simulink model "SVPWM"  (R2023a)
settings: Solver=VariableStepAuto  StartTime=0.0  StopTime=1  MaxStep=0.0001  RelTol=1e-3
libraries: spsMosfetLib x6, spspowerguiLib x2, spsThreePhaseVIMeasurementLib x2, spsDCVoltageSourceLib x1, spsGroundLib x1, spsThreePhaseSeriesRLCBranchLib x1, spsTriangleGeneratorLib x1
settings Model: Creator=patri  LastModifiedBy=patri

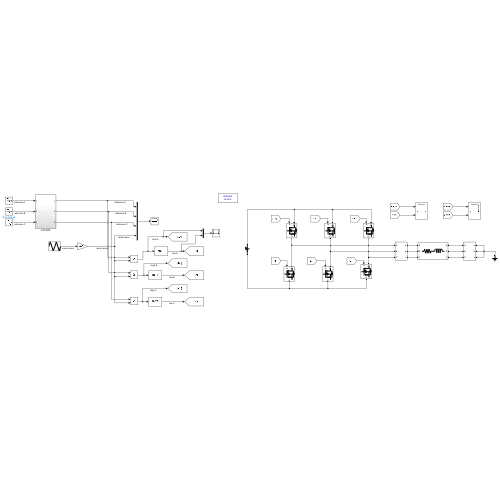
[thumbnail: Simulink's stored preview of the top-level diagram]
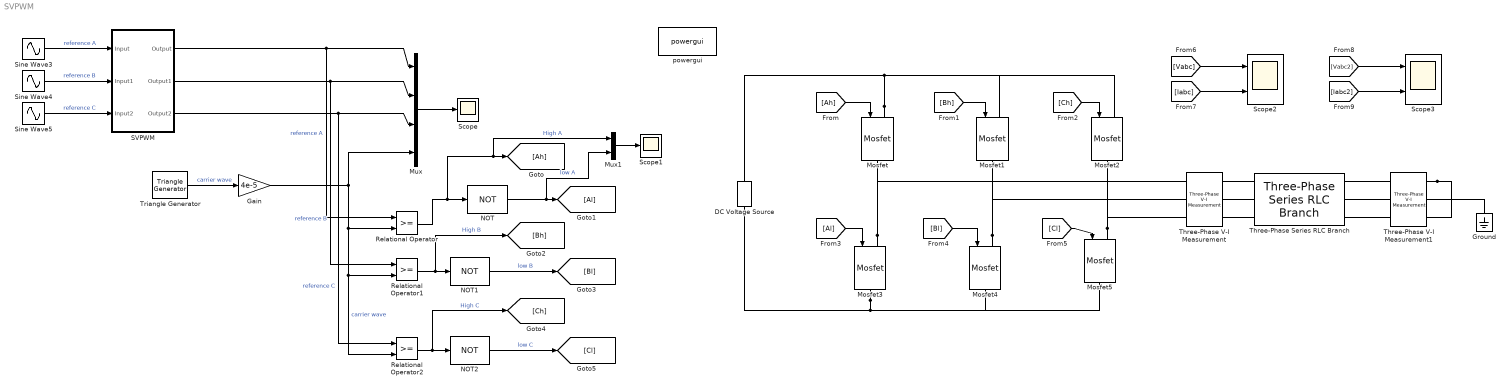
== system SVPWM ==
  DC Voltage Source : spsDCVoltageSourceLib/DC Voltage Source  Amplitude=100  Measurements=None
  Gain : Gain  Gain=4e-5
  Ground : spsGroundLib/Ground  LConnTagsString=a
  Mosfet{,1..5} (6 alike) : spsMosfetLib/Mosfet  Ron=0.1  Lon=0  Rd=0.01  Vfd=0  IC=0  Rs=1e5  Cs=inf  Measurements=off
  Mux : Mux
  Mux1 : Mux  Inputs=2
  NOT : Logic  Operator=NOT  AllPortsSameDT=off  OutDataTypeStr=boolean
  NOT1 : Logic  Operator=NOT  AllPortsSameDT=off  OutDataTypeStr=boolean
  NOT2 : Logic  Operator=NOT  AllPortsSameDT=off  OutDataTypeStr=boolean
  Relational Operator : RelationalOperator  OutDataTypeStr=boolean  RndMeth=Simplest  InputSameDT=off
  Relational Operator1 : RelationalOperator  OutDataTypeStr=boolean  RndMeth=Simplest  InputSameDT=off
  Relational Operator2 : RelationalOperator  OutDataTypeStr=boolean  RndMeth=Simplest  InputSameDT=off
  SVPWM : Subsystem
  Scope : Scope
  Scope1 : Scope
  Scope2 : Scope  NumInputPorts=2
  Scope3 : Scope  NumInputPorts=2
  Sine Wave3 : Sin  Frequency=2*pi*50  SampleTime=0
  Sine Wave4 : Sin  Frequency=2*pi*50  Phase=2*pi/3  SampleTime=0
  Sine Wave5 : Sin  Frequency=2*pi*50  Phase=4*pi/3  SampleTime=0
  Three-Phase Series RLC Branch : spsThreePhaseSeriesRLCBranchLib/Three-Phase Series RLC Branch  LConnTagsString=A|B|C  RConnTagsString=A|B|C  BranchType=RL  Resistance=1  Inductance=1e-3  Capacitance=1e-6  Measurements=None
  Three-Phase V-I Measurement : spsThreePhaseVIMeasurementLib/Three-Phase V-I Measurement  VoltageMeasurement=phase-to-ground  SetLabelV=on  LabelV=Vabc  Vpu=off  VpuLL=off  CurrentMeasurement=yes  SetLabelI=on  LabelI=Iabc  Ipu=off  Pbase=100e6  Vbase=500e3  OutputType=Complex  PhasorSimulation=off  PSBequivalent=0
  Three-Phase V-I Measurement1 : spsThreePhaseVIMeasurementLib/Three-Phase V-I Measurement  VoltageMeasurement=phase-to-ground  SetLabelV=on  LabelV=Vabc2  Vpu=off  VpuLL=off  CurrentMeasurement=yes  SetLabelI=on  LabelI=Iabc2  Ipu=off  Pbase=100e6  Vbase=500e3  OutputType=Complex  PhasorSimulation=off  PSBequivalent=0
  Triangle Generator : spsTriangleGeneratorLib/Triangle Generator  Freq=10e3  Phase=90  Ts=0
  powergui : spspowerguiLib/powergui  Priority=1  SimulationMode=Discrete  SampleTime=1e-6  frequency=60  Iterations=50  frequencyindice=0  Pbase=100e6  ErrMax=1e-4  UnitsV=kV  UnitsW=MW  buscounter=0  FunctionMessages=off  echomessages=off  EnableUseOfTLC=off  CurrentSourceSwitches=off  DisableSnubberDevices=off  DisableRonSwitches=off  DisableVfSwitches=off  DisplayEquations=off  AutomaticDiscreteSolvers=off  SolverType=Tustin/Backward Euler (TBE)  Interpol=off  ExternalGateDelay=off  methode=off  Ts=100  x0status=blocks  SPID=on  SwTol=0  HookPort=off  NonlinearTolerance=1e-4  nMaxIteration=100  ContinueOnMaxIteration=off  RestoreLinks=warning  ResistiveCurrentMeasurement=off  Frange=[0:2:500]  Ylog=off  Xlog=on  ShowGrid=off  save=off  variable=ZData  structure=0  ZoomFFT=off  StartTime=0.0  cycles=1  DisplayStyle=1  fundamental=60  FreqAxis=off  MaxFrequency=1000  frequencyindicesteady=1  RmsSteady=1  display=off
  wires:
  [Vabc2] -> Scope3/1
  [Al] -> Mosfet3/1
  [Vabc] -> Scope2/1
  [Cl] -> Mosfet5/1
  [Bh] -> Mosfet1/1
  [Ch] -> Mosfet2/1
  [Bl] -> Mosfet4/1
  [Iabc] -> Scope2/2
  [Iabc2] -> Scope3/2
  [Ah] -> Mosfet/1
  Sine Wave3/1 -> SVPWM/1(Input)  "reference A"
  Sine Wave4/1 -> SVPWM/2(Input1)  "reference B"
  Sine Wave5/1 -> SVPWM/3(Input2)  "reference C"
  Mux/1 -> Scope/1
  Mux1/1 -> Scope1/1
  NOT1/1 -> [Bl]  "low B"
  NOT/1 -> Mux1/2, [Al]  "low A"
  Relational Operator2/1 -> [Ch], NOT2/1  "High C"
  NOT2/1 -> [Cl]  "low C"
  Triangle Generator/1 -> Gain/1  "carrier wave"
  Relational Operator1/1 -> [Bh], NOT1/1  "High B"
  Relational Operator/1 -> Mux1/1, [Ah], NOT/1  "High A"
  SVPWM/3(Output2) -> Relational Operator2/1, Mux/3  "reference C"
  SVPWM/2(Output1) -> Relational Operator1/1, Mux/2  "reference B"
  SVPWM/1(Output) -> Relational Operator/1, Mux/1  "reference A"
  Gain/1 -> Relational Operator2/2, Relational Operator1/2, Relational Operator/2, Mux/4  "carrier wave"
  connections:
  Mosfet3/RConn1 -- DC Voltage Source/LConn1 -- Mosfet4/RConn1 -- Mosfet5/RConn1
  Three-Phase V-I Measurement1/RConn1 -- Three-Phase V-I Measurement1/RConn2 -- Ground/LConn1 -- Three-Phase V-I Measurement1/RConn3
  Mosfet/LConn1 -- DC Voltage Source/RConn1 -- Mosfet2/LConn1 -- Mosfet1/LConn1
  Mosfet4/LConn1 -- Mosfet1/RConn1 -- Three-Phase V-I Measurement/LConn2
  Mosfet3/LConn1 -- Mosfet/RConn1 -- Three-Phase V-I Measurement/LConn1
  Mosfet5/LConn1 -- Mosfet2/RConn1 -- Three-Phase V-I Measurement/LConn3
  Three-Phase V-I Measurement/RConn1 -- Three-Phase Series RLC Branch/LConn1
  Three-Phase V-I Measurement1/LConn3 -- Three-Phase Series RLC Branch/RConn3
  Three-Phase V-I Measurement1/LConn1 -- Three-Phase Series RLC Branch/RConn1
  Three-Phase Series RLC Branch/LConn2 -- Three-Phase V-I Measurement/RConn2
  Three-Phase V-I Measurement/RConn3 -- Three-Phase Series RLC Branch/LConn3
  Three-Phase V-I Measurement1/LConn2 -- Three-Phase Series RLC Branch/RConn2

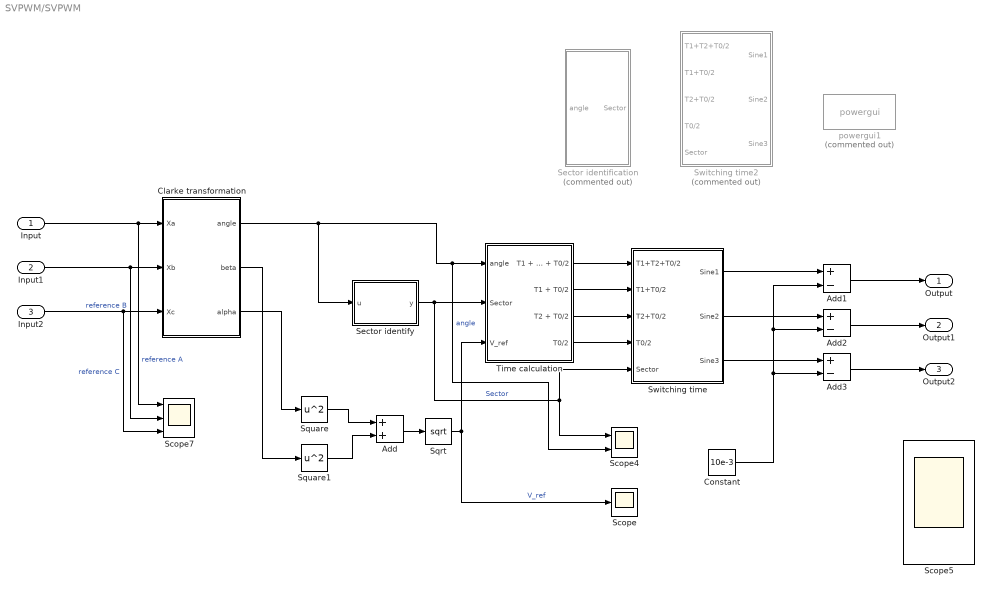
== system SVPWM/SVPWM ==
  Input : Inport
  Input1 : Inport  Port=2
  Input2 : Inport  Port=3
  Add : Sum
  Add1 : Sum  Inputs=+-
  Add2 : Sum  Inputs=+-
  Add3 : Sum  Inputs=+-
  Clarke transformation : Subsystem
  Constant : Constant  Value=10e-3
  Scope : Scope
  Scope4 : Scope  NumInputPorts=2
  Scope5 : Scope  NumInputPorts=3
  Scope7 : Scope  NumInputPorts=3
  Sector identification : Subsystem  Commented=on
  Sector identify : MATLAB Function  TreatAsAtomicUnit=on
  Sqrt : Sqrt
  Square : Math  Operator=square
  Square1 : Math  Operator=square
  Switching time : Subsystem
  Switching time2 : Subsystem  Commented=on
  Time calculation : Subsystem
  powergui1 : spspowerguiLib/powergui  Priority=1  Commented=on  SimulationMode=Continuous  SampleTime=50e-6  frequency=60  Iterations=50  frequencyindice=60  Pbase=100e6  ErrMax=1e-4  UnitsV=kV  UnitsW=MW  buscounter=0  FunctionMessages=off  echomessages=off  EnableUseOfTLC=off  CurrentSourceSwitches=off  DisableSnubberDevices=off  DisableRonSwitches=off  DisableVfSwitches=off  DisplayEquations=off  AutomaticDiscreteSolvers=off  SolverType=Tustin/Backward Euler (TBE)  Interpol=off  ExternalGateDelay=off  methode=off  Ts=100  x0status=blocks  SPID=on  SwTol=0  HookPort=off  NonlinearTolerance=1e-4  nMaxIteration=100  ContinueOnMaxIteration=off  RestoreLinks=warning  ResistiveCurrentMeasurement=off  Frange=[0:2:500]  Ylog=off  Xlog=on  ShowGrid=off  save=off  variable=ZData  structure=0  ZoomFFT=off  StartTime=0.0  cycles=1  DisplayStyle=1  fundamental=60  FreqAxis=off  MaxFrequency=1000  frequencyindicesteady=1  RmsSteady=1  display=off
  Output : Outport
  Output1 : Outport  Port=2
  Output2 : Outport  Port=3
  wires:
  Sector identify/1(y) -> Switching time/5(Sector), Scope4/1, Time calculation/2(Sector)  "Sector"
  Sqrt/1 -> Scope/1, Time calculation/3(V_ref)  "V_ref"
  Input1/1 -> Scope7/2, Clarke transformation/2(Xb)  "reference B"
  Time calculation/3(T2 + T0/2) -> Switching time/3(T2+T0/2)
  Square/1 -> Add/1
  Square1/1 -> Add/2
  Time calculation/1(T1 + T2 + T0/2) -> Switching time/1(T1+T2+T0/2)
  Time calculation/2(T1 + T0/2) -> Switching time/2(T1+T0/2)
  Input/1 -> Scope7/1, Clarke transformation/1(Xa)  "reference A"
  Input2/1 -> Scope7/3, Clarke transformation/3(Xc)  "reference C"
  Clarke transformation/1(angle) -> Scope4/2, Time calculation/1(angle), Sector identify/1(u)  "angle"
  Time calculation/4(T0/2) -> Switching time/4(T0/2)
  Clarke transformation/2(beta) -> Square1/1
  Clarke transformation/3(alpha) -> Square/1
  Add/1 -> Sqrt/1
  Constant/1 -> Add3/2, Add2/2, Add1/2
  Switching time/1(Sine1) -> Add1/1
  Add1/1 -> Output/1
  Switching time/2(Sine2) -> Add2/1
  Switching time/3(Sine3) -> Add3/1
  Add2/1 -> Output1/1
  Add3/1 -> Output2/1

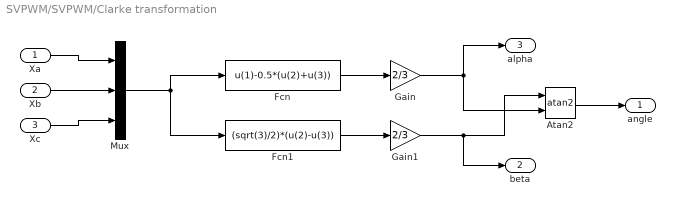
== system SVPWM/SVPWM/Clarke transformation ==
  Xa : Inport
  Xb : Inport  Port=2
  Xc : Inport  Port=3
  Atan2 : Trigonometry  Operator=atan2
  Fcn : Fcn  Expr=u(1)-0.5*(u(2)+u(3))
  Fcn1 : Fcn  Expr=(sqrt(3)/2)*(u(2)-u(3))
  Gain : Gain  Gain=2/3
  Gain1 : Gain  Gain=2/3
  Mux : Mux  Inputs=3
  angle : Outport
  beta : Outport  Port=2
  alpha : Outport  Port=3
  wires:
  Xc/1 -> Mux/3
  Xb/1 -> Mux/2
  Xa/1 -> Mux/1
  Mux/1 -> Fcn1/1, Fcn/1
  Fcn/1 -> Gain/1
  Fcn1/1 -> Gain1/1
  Gain/1 -> Atan2/2, alpha/1
  Gain1/1 -> Atan2/1, beta/1
  Atan2/1 -> angle/1

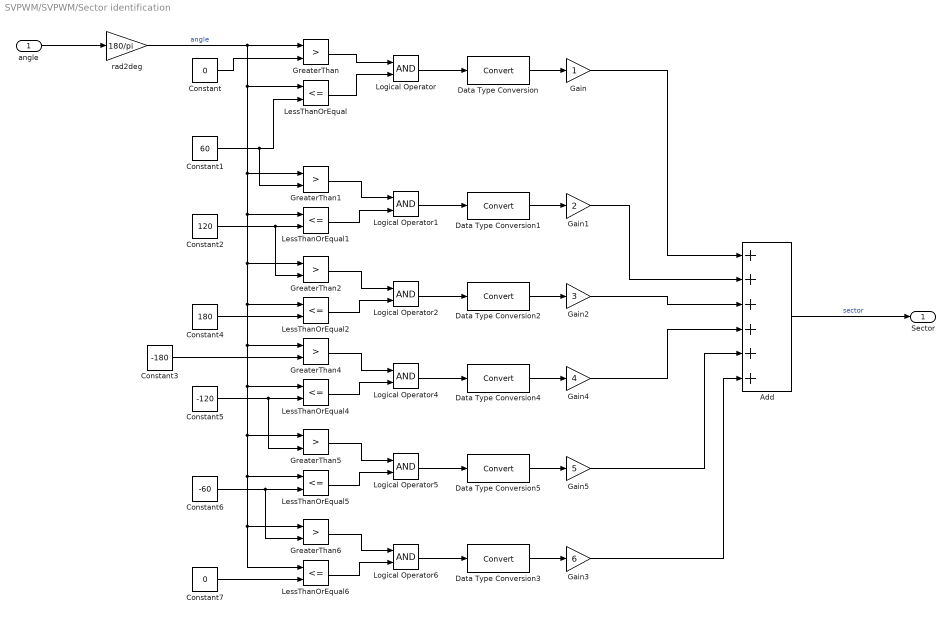
== system SVPWM/SVPWM/Sector identification ==
  angle : Inport
  Add : Sum  Inputs=++++++
  Constant : Constant  Value=0
  Constant1 : Constant  Value=60
  Constant2 : Constant  Value=120
  Constant3 : Constant  Value=-180
  Constant4 : Constant  Value=180
  Constant5 : Constant  Value=-120
  Constant6 : Constant  Value=-60
  Constant7 : Constant  Value=0
  Data Type Conversion{,1..5} (6 alike) : DataTypeConversion  SaturateOnIntegerOverflow=off  RndMeth=Floor
  Gain : Gain
  Gain1 : Gain  Gain=2
  Gain2 : Gain  Gain=3
  Gain3 : Gain  Gain=6
  Gain4 : Gain  Gain=4
  Gain5 : Gain  Gain=5
  GreaterThan{,1..2,4..6} (6 alike) : RelationalOperator  Operator=>  OutDataTypeStr=boolean  RndMeth=Simplest  InputSameDT=off
  LessThanOrEqual{,1..2,4..6} (6 alike) : RelationalOperator  Operator=<=  OutDataTypeStr=boolean  RndMeth=Simplest  InputSameDT=off
  Logical Operator{,1..2,4..6} (6 alike) : Logic  AllPortsSameDT=off  OutDataTypeStr=boolean
  rad2deg : Gain  Gain=180/pi
  Sector : Outport
  wires:
  Data Type Conversion1/1 -> Gain1/1
  LessThanOrEqual6/1 -> Logical Operator6/2
  Constant1/1 -> GreaterThan1/2, LessThanOrEqual/2
  LessThanOrEqual2/1 -> Logical Operator2/2
  LessThanOrEqual4/1 -> Logical Operator4/2
  LessThanOrEqual5/1 -> Logical Operator5/2
  Constant2/1 -> GreaterThan2/2, LessThanOrEqual1/2
  LessThanOrEqual/1 -> Logical Operator/2
  Constant7/1 -> LessThanOrEqual6/2
  Constant6/1 -> GreaterThan6/2, LessThanOrEqual5/2
  LessThanOrEqual1/1 -> Logical Operator1/2
  Constant4/1 -> LessThanOrEqual2/2
  GreaterThan5/1 -> Logical Operator5/1
  GreaterThan6/1 -> Logical Operator6/1
  GreaterThan4/1 -> Logical Operator4/1
  Data Type Conversion/1 -> Gain/1
  Data Type Conversion3/1 -> Gain3/1
  Logical Operator6/1 -> Data Type Conversion3/1
  Data Type Conversion4/1 -> Gain4/1
  Logical Operator2/1 -> Data Type Conversion2/1
  Constant5/1 -> GreaterThan5/2, LessThanOrEqual4/2
  Logical Operator4/1 -> Data Type Conversion4/1
  GreaterThan/1 -> Logical Operator/1
  Constant/1 -> GreaterThan/2
  GreaterThan1/1 -> Logical Operator1/1
  Logical Operator5/1 -> Data Type Conversion5/1
  Logical Operator/1 -> Data Type Conversion/1
  GreaterThan2/1 -> Logical Operator2/1
  Data Type Conversion5/1 -> Gain5/1
  Data Type Conversion2/1 -> Gain2/1
  Constant3/1 -> GreaterThan4/2
  Logical Operator1/1 -> Data Type Conversion1/1
  Gain/1 -> Add/1
  Gain1/1 -> Add/2
  Gain2/1 -> Add/3
  Gain4/1 -> Add/4
  Gain5/1 -> Add/5
  Gain3/1 -> Add/6
  Add/1 -> Sector/1  "sector"
  angle/1 -> rad2deg/1
  rad2deg/1 -> LessThanOrEqual6/1, GreaterThan6/1, LessThanOrEqual5/1, GreaterThan5/1, LessThanOrEqual4/1, GreaterThan4/1, LessThanOrEqual2/1, GreaterThan2/1, LessThanOrEqual1/1, GreaterThan1/1, LessThanOrEqual/1, GreaterThan/1  "angle"

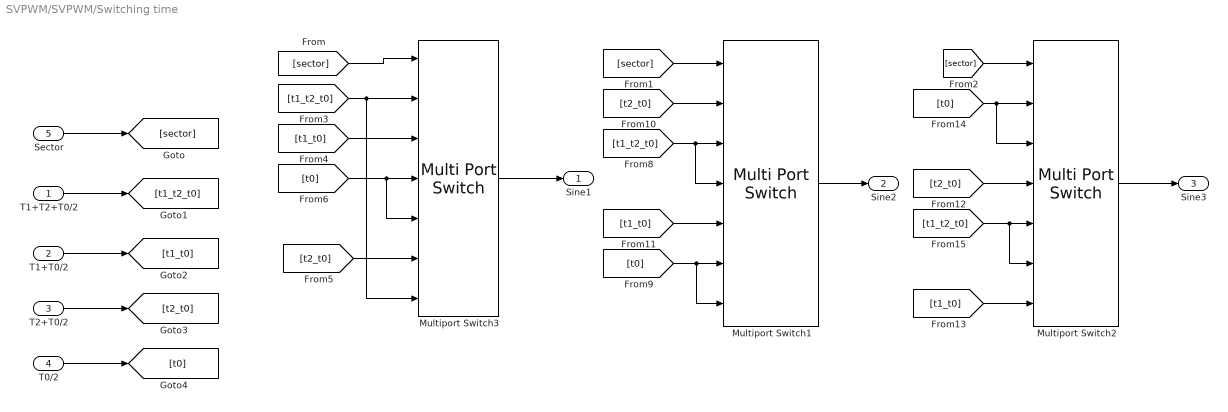
== system SVPWM/SVPWM/Switching time ==
  T1+T2+T0/2 : Inport
  T1+T0/2 : Inport  Port=2
  T2+T0/2 : Inport  Port=3
  T0/2 : Inport  Port=4
  Sector : Inport  Port=5
  Multiport Switch1 : MultiPortSwitch  Inputs=6  DiagnosticForDefault=Warning  SaturateOnIntegerOverflow=off  InputSameDT=off
  Multiport Switch2 : MultiPortSwitch  Inputs=6  DiagnosticForDefault=Warning  SaturateOnIntegerOverflow=off  InputSameDT=off
  Multiport Switch3 : MultiPortSwitch  Inputs=6  DiagnosticForDefault=Warning  SaturateOnIntegerOverflow=off  InputSameDT=off
  Sine1 : Outport
  Sine2 : Outport  Port=2
  Sine3 : Outport  Port=3
  wires:
  Multiport Switch3/1 -> Sine1/1
  Sector/1 -> [sector]
  T1+T2+T0/2/1 -> [t1_t2_t0]
  [sector] -> Multiport Switch3/1
  [sector] -> Multiport Switch1/1
  [sector] -> Multiport Switch2/1
  Multiport Switch1/1 -> Sine2/1
  Multiport Switch2/1 -> Sine3/1
  T1+T0/2/1 -> [t1_t0]
  T2+T0/2/1 -> [t2_t0]
  T0/2/1 -> [t0]
  [t1_t2_t0] -> Multiport Switch3/7, Multiport Switch3/2
  [t1_t2_t0] -> Multiport Switch1/4, Multiport Switch1/3
  [t1_t2_t0] -> Multiport Switch2/6, Multiport Switch2/5
  [t1_t0] -> Multiport Switch3/3
  [t0] -> Multiport Switch3/5, Multiport Switch3/4
  [t2_t0] -> Multiport Switch3/6
  [t2_t0] -> Multiport Switch1/2
  [t1_t0] -> Multiport Switch1/5
  [t0] -> Multiport Switch1/7, Multiport Switch1/6
  [t1_t0] -> Multiport Switch2/7
  [t2_t0] -> Multiport Switch2/4
  [t0] -> Multiport Switch2/3, Multiport Switch2/2

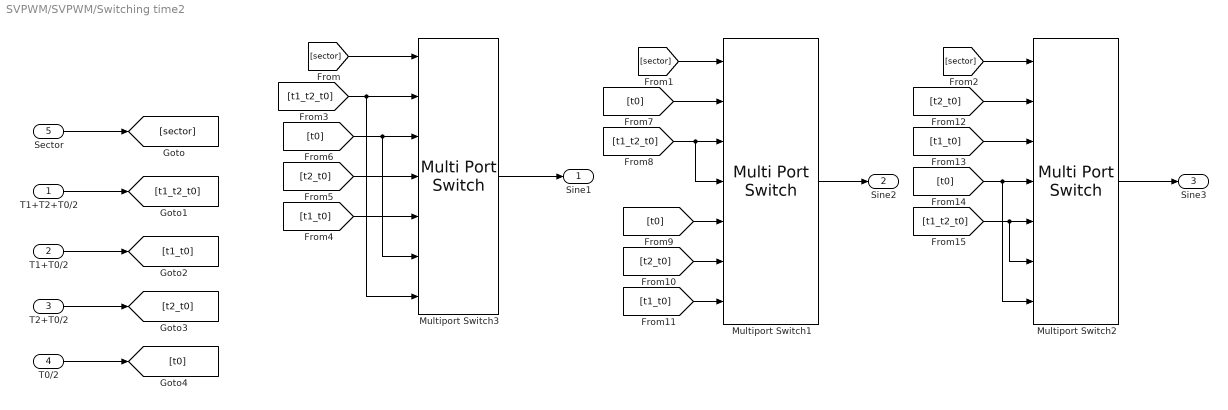
== system SVPWM/SVPWM/Switching time2 ==
  T1+T2+T0/2 : Inport
  T1+T0/2 : Inport  Port=2
  T2+T0/2 : Inport  Port=3
  T0/2 : Inport  Port=4
  Sector : Inport  Port=5
  Multiport Switch1 : MultiPortSwitch  Inputs=6  SaturateOnIntegerOverflow=off  InputSameDT=off
  Multiport Switch2 : MultiPortSwitch  Inputs=6  SaturateOnIntegerOverflow=off  InputSameDT=off
  Multiport Switch3 : MultiPortSwitch  Inputs=6  SaturateOnIntegerOverflow=off  InputSameDT=off
  Sine1 : Outport
  Sine2 : Outport  Port=2
  Sine3 : Outport  Port=3
  wires:
  Multiport Switch3/1 -> Sine1/1
  Sector/1 -> [sector]
  T1+T2+T0/2/1 -> [t1_t2_t0]
  [sector] -> Multiport Switch3/1
  [sector] -> Multiport Switch1/1
  [sector] -> Multiport Switch2/1
  Multiport Switch1/1 -> Sine2/1
  Multiport Switch2/1 -> Sine3/1
  T1+T0/2/1 -> [t1_t0]
  T2+T0/2/1 -> [t2_t0]
  T0/2/1 -> [t0]
  [t1_t2_t0] -> Multiport Switch3/7, Multiport Switch3/2
  [t0] -> Multiport Switch3/6, Multiport Switch3/3
  [t2_t0] -> Multiport Switch3/4
  [t1_t0] -> Multiport Switch3/5
  [t0] -> Multiport Switch1/2
  [t1_t2_t0] -> Multiport Switch1/4, Multiport Switch1/3
  [t0] -> Multiport Switch1/5
  [t2_t0] -> Multiport Switch1/6
  [t1_t0] -> Multiport Switch1/7
  [t2_t0] -> Multiport Switch2/2
  [t1_t0] -> Multiport Switch2/3
  [t0] -> Multiport Switch2/4, Multiport Switch2/7
  [t1_t2_t0] -> Multiport Switch2/6, Multiport Switch2/5

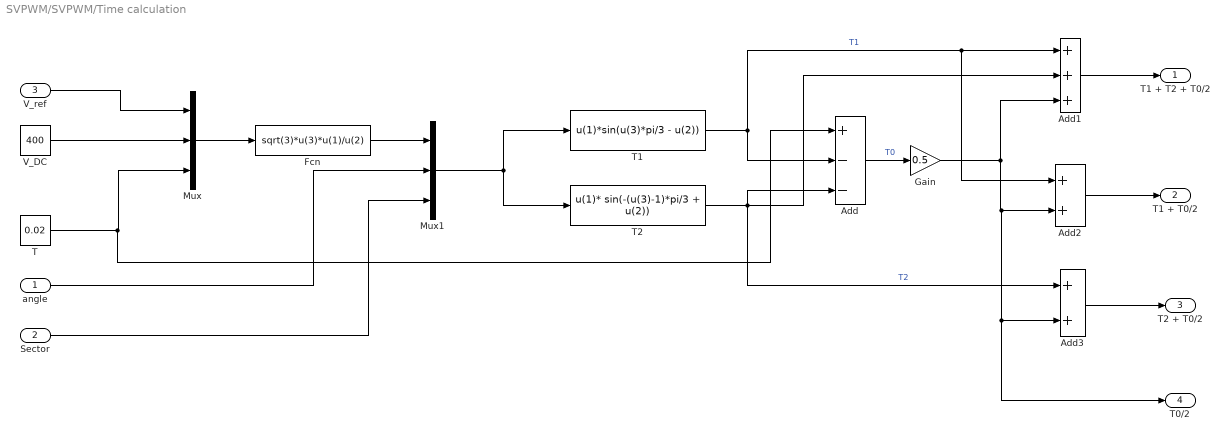
== system SVPWM/SVPWM/Time calculation ==
  angle : Inport
  Sector : Inport  Port=2
  V_ref : Inport  Port=3
  Add : Sum  Inputs=+--
  Add1 : Sum  Inputs=+++
  Add2 : Sum
  Add3 : Sum
  Fcn : Fcn  Expr=sqrt(3)*u(3)*u(1)/u(2)
  Gain : Gain  Gain=0.5
  Mux : Mux  Inputs=3
  Mux1 : Mux  Inputs=3
  T : Constant  Value=0.02
  T1 : Fcn  Expr=u(1)*sin(u(3)*pi/3 - u(2))
  T2 : Fcn  Expr=u(1)* sin(-(u(3)-1)*pi/3 + u(2))
  V_DC : Constant  Value=400
  T1 + T2 + T0/2 : Outport
  T1 + T0/2 : Outport  Port=2
  T2 + T0/2 : Outport  Port=3
  T0/2 : Outport  Port=4
  wires:
  Mux/1 -> Fcn/1
  V_DC/1 -> Mux/2
  T/1 -> Add/1, Mux/3
  Fcn/1 -> Mux1/1
  angle/1 -> Mux1/2
  Sector/1 -> Mux1/3
  Mux1/1 -> T2/1, T1/1
  T1/1 -> Add2/1, Add1/1, Add/2  "T1"
  T2/1 -> Add3/1, Add1/2, Add/3  "T2"
  Add/1 -> Gain/1  "T0"
  Add1/1 -> T1 + T2 + T0/2/1
  Gain/1 -> T0/2/1, Add3/2, Add2/2, Add1/3
  Add2/1 -> T1 + T0/2/1
  Add3/1 -> T2 + T0/2/1
  V_ref/1 -> Mux/1

== matlab function SVPWM/Sector identify ==
  data: u input; y output
function y = fcn(u)

u = u* (180/pi);         % rad to degrees

if (u>0) && (u<=60)
    u=1;
elseif (u>60) && (u<=120)
    u=2;
elseif (u>120) && (u<=180)
    u=3;
elseif (u>-180) && (u<=-120)
    u=4;
elseif (u>-120) && (u<=-60)
    u=5;
elseif (u>-60) && (u<=0)
    u=6;
else
    u=0;
end
y = u;
